simulink model "CoolingSystemR2024a_testingl"  (R2024a)
settings: Solver=ode1be  StartTime=0.0  StopTime=60*60  RelTol=1e-3
values from neighbouring files (symbols this model uses):
  cp = 4190    [parameters.m]
  M_B = 10000    [parameters.m]
  M_E = 2000    [parameters.m]
  M_MIX = 20    [parameters.m]
  mdot_ini = 30    [parameters.m]
  T_in = 60    [parameters.m]
  T_ini = 60    [parameters.m]
libraries: slpidlib x1
settings Model: ExtModeTrigDuration=100  Creator=mikman2  LastModifiedBy=ojklem
settings DataIOCC: StateSaveName=tmp_raccel_xout
settings OptimizationCC: EfficientMapNaN2IntZero=off
settings DebuggingCC: AlgebraicLoopMsg=error
settings RTWCC: CustomBLASCallback=coder.internal.blas.MATLABBLASCallback
settings CodeAppCC: GenerateComments=off  SimulinkBlockComments=off

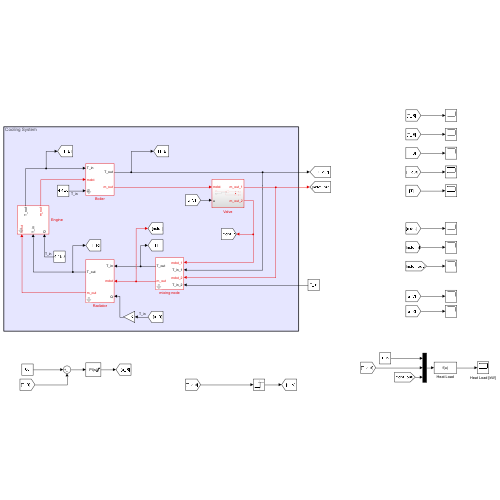
[thumbnail: Simulink's stored preview of the top-level diagram]
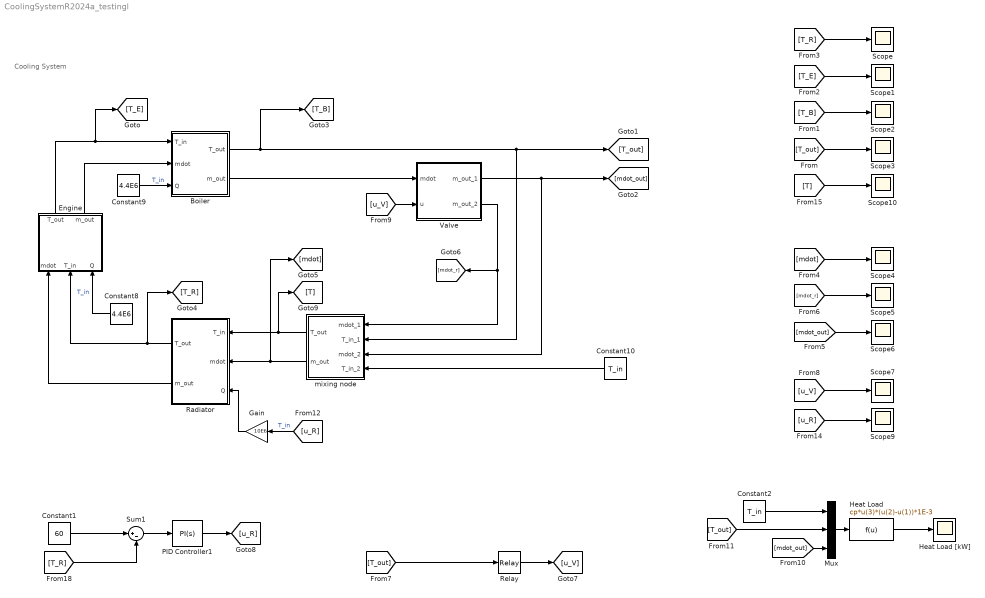
== system CoolingSystemR2024a_testingl ==
  note: Cooling System
  Boiler : Subsystem  mask{M=M_B, cp=cp}
      mask prompts: M "Mass [kg]"; cp "Specific heat capacity [J/kg/K]"
  Constant1 : Constant  Value=60
  Constant10 : Constant  Value=T_in
  Constant2 : Constant  Value=T_in
  Constant8 : Constant  Value=4.4E6
  Constant9 : Constant  Value=4.4E6
  Engine : Subsystem  mask{M=M_E, cp=cp}
      mask prompts: M "Mass [kg]"; cp "Specific heat capacity [J/kg/K]"
  Gain : Gain  Gain=10E6
  Heat Load : Fcn  Expr=cp*u(3)*(u(2)-u(1))*1E-3
  Heat Load [kW] : Scope
  Mux : Mux  Inputs=3
  PID Controller1 : slpidlib/PID Controller  Controller=PI  Form=Ideal  TimeDomain=Continuous-time  UseExternalTs=off  SampleTime=-1  IntegratorMethod=Forward Euler  FilterMethod=Forward Euler  ControllerParametersSource=internal  P=-0.05  I=1/120  UseKiTs=off  D=0  UseExternalDerivativeSource=off  N=100  UseFilter=on  TunerSelectOption=Transfer Function Based (PID Tuner App)  InitialConditionSource=internal  InitialConditionForIntegrator=0  InitialConditionForFilter=0  DifferentiatorICPrevScaledInput=0  ExternalReset=none  TrackingMode=off  Kt=1  LimitOutput=on  SatLimitsSource=internal  UpperSaturationLimit=1  LowerSaturationLimit=0  LinearizeAsGain=on  AntiWindupMode=none  Kb=1  LimitIntegrator=off  UpperIntegratorSaturationLimit=inf  LowerIntegratorSaturationLimit=-inf  POutMin=[]  POutMax=[]  IOutMin=[]  IOutMax=[]  DOutMin=[]  DOutMax=[]  NOutMin=[]  NOutMax=[]  SumOutMin=[]  SumOutMax=[]  SaturationOutMin=[]  SaturationOutMax=[]  PParamMin=[]  PParamMax=[]  IParamMin=[]  IParamMax=[]  DParamMin=[]  DParamMax=[]  NParamMin=[]  NParamMax=[]  KbParamMin=[]  KbParamMax=[]  KtParamMin=[]  KtParamMax=[]  KbOutMin=[]  KbOutMax=[]  KtOutMin=[]  KtOutMax=[]  IntegratorOutMin=[]  IntegratorOutMax=[]  FilterOutMin=[]  FilterOutMax=[]  SumI1OutMin=[]  SumI1OutMax=[]  SumI2OutMin=[]  SumI2OutMax=[]  SumI3OutMin=[]  SumI3OutMax=[]  SumI4OutMin=[]  SumI4OutMax=[]  SumDOutMin=[]  SumDOutMax=[]  DifferentiatorOutMin=[]  DifferentiatorOutMax=[]  FilterDiffOutCoefMin=[]  FilterDiffOutCoefMax=[]  ReciprocalOutMin=[]  ReciprocalOutMax=[]  SumDenOutMin=[]  SumDenOutMax=[]  SumNumOutMin=[]  SumNumOutMax=[]  DivideOutMin=[]  DivideOutMax=[]  UdiffTsProdOutMin=[]  UdiffTsProdOutMax=[]  NTsProdOutMin=[]  NTsProdOutMax=[]  UintegralTsProdOutMin=[]  UintegralTsProdOutMax=[]  UngainTsProdOutMin=[]  UngainTsProdOutMax=[]  ClampingZeroOutDataTypeStr=Inherit: Inherit via back propagation  ClampingZeroOutMin=[]  ClampingZeroOutMax=[]  FilterDenConstantOutDataTypeStr=Inherit: Inherit via back propagation  FilterDenConstantOutMin=[]  FilterDenConstantOutMax=[]  PCopyOutDataTypeStr=Inherit: Inherit via back propagation  PCopyOutMin=[]  PCopyOutMax=[]  NCopyOutDataTypeStr=Inherit: Inherit via back propagation  NCopyOutMin=[]  NCopyOutMax=[]  IntegratorContinuousStateAttributes=''  IntegratorStateMustResolveToSignalObject=off  IntegratorRTWStateStorageClass=Auto  FilterContinuousStateAttributes=''  FilterStateMustResolveToSignalObject=off  FilterRTWStateStorageClass=Auto  ParallelPVariant=Passthrough  IdealPVariant=InternalParameters  IVariant=InternalParameters  DVariant=Disabled  IntegratorVariant=Continuous  SatVariant=Enabled  AWVariant=Passthrough  PCopyVariant=Disabled  TRVariant=Disabled  FdbkBlocksVariant=Forward  IdealPFdbkVariant=Disabled  SatFdbkVariant=Disabled  DerivativeFilterVariant=Disabled  NVariant=Disabled  NCopyVariant=Disabled_SignalSpec  FilterICVariant=Disabled  IntegratorICVariant=InternalICs  ExternalResetVariant=Disabled  TRSumVariant=Passthrough  SumFdbkVariant=Disabled  SumVariant=Sum_PI  TsampFilterVariant=InternalTs  TsampNgainVariant=Passthrough  TsampIntegralVariant=Disabled_SignalSpec  ExternalSaturationOutDataTypeStr=Inherit: Same as second input  DerivativeSourceVariant=Disabled
  Radiator : Subsystem  mask{M=M_E, cp=cp}
      mask prompts: M "Mass [kg]"; cp "Specific heat capacity [J/kg/K]"
  Relay : Relay  OnSwitchValue=125  OffSwitchValue=0
  Scope{,1..7,9..10} (10 alike) : Scope
  Sum1 : Sum  Inputs=|+-
  Valve : Subsystem
  mixing node : Subsystem  mask{M=M_MIX, cp=cp}
      mask prompts: M "Mass [kg]"; cp "Specific heat capacity [J/kg/K]"
  wires:
  mixing node/1(T_out) -> [T], Radiator/1(T_in)
  mixing node/2(m_out) -> [mdot], Radiator/2(mdot)
  [u_R] -> Gain/1  "T_in"
  Radiator/2(m_out) -> Engine/1(mdot)
  Radiator/1(T_out) -> [T_R], Engine/2(T_in)
  Constant8/1 -> Engine/3(Q)  "T_in"
  Engine/1(T_out) -> Boiler/1(T_in), [T_E]
  Engine/2(m_out) -> Boiler/2(mdot)
  Constant9/1 -> Boiler/3(Q)  "T_in"
  Boiler/1(T_out) -> [T_B], mixing node/2(T_in_1), [T_out]
  Valve/1(m_out_1) -> [mdot_out], mixing node/3(mdot_2)
  Constant10/1 -> mixing node/4(T_in_2)
  Valve/2(m_out_2) -> mixing node/1(mdot_1), [mdot_r]
  Boiler/2(m_out) -> Valve/1(mdot)
  [u_V] -> Valve/2(u)
  [T_R] -> Scope/1
  [T_B] -> Scope2/1
  [T_E] -> Scope1/1
  [T_out] -> Scope3/1
  [mdot] -> Scope4/1
  [mdot_r] -> Scope5/1
  [mdot_out] -> Scope6/1
  [u_V] -> Scope7/1
  Gain/1 -> Radiator/3(Q)
  [u_R] -> Scope9/1
  [T] -> Scope10/1
  [T_out] -> Relay/1
  Relay/1 -> [u_V]
  Mux/1 -> Heat Load/1
  [mdot_out] -> Mux/3
  Constant2/1 -> Mux/1
  [T_out] -> Mux/2
  Heat Load/1 -> Heat Load [kW]/1
  Sum1/1 -> PID Controller1/1
  [T_R] -> Sum1/2
  Constant1/1 -> Sum1/1
  PID Controller1/1 -> [u_R]

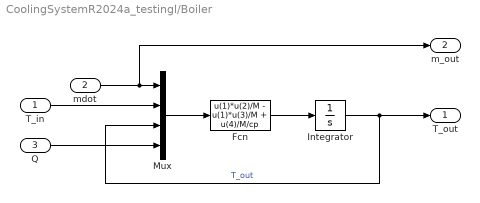
== system CoolingSystemR2024a_testingl/Boiler ==
  T_in : Inport
  mdot : Inport  Port=2
  Q : Inport  Port=3
  Fcn : Fcn  Expr=u(1)*u(2)/M - u(1)*u(3)/M + u(4)/M/cp
  Integrator : Integrator  InitialCondition=T_ini
  Mux : Mux
  T_out : Outport
  m_out : Outport  Port=2
  wires:
  Q/1 -> Mux/4
  T_in/1 -> Mux/2
  Mux/1 -> Fcn/1
  Fcn/1 -> Integrator/1
  mdot/1 -> m_out/1, Mux/1
  Integrator/1 -> T_out/1, Mux/3  "T_out"

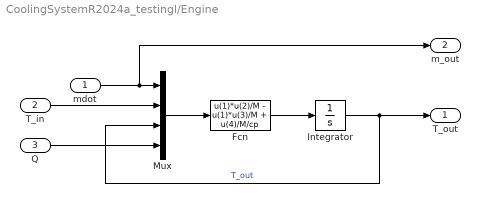
== system CoolingSystemR2024a_testingl/Engine ==
  mdot : Inport
  T_in : Inport  Port=2
  Q : Inport  Port=3
  Fcn : Fcn  Expr=u(1)*u(2)/M - u(1)*u(3)/M + u(4)/M/cp
  Integrator : Integrator  InitialCondition=T_ini
  Mux : Mux
  T_out : Outport
  m_out : Outport  Port=2
  wires:
  Integrator/1 -> Mux/3, T_out/1  "T_out"
  mdot/1 -> Mux/1, m_out/1
  Fcn/1 -> Integrator/1
  Mux/1 -> Fcn/1
  T_in/1 -> Mux/2
  Q/1 -> Mux/4

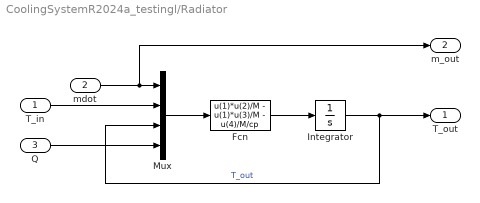
== system CoolingSystemR2024a_testingl/Radiator ==
  T_in : Inport
  mdot : Inport  Port=2
  Q : Inport  Port=3
  Fcn : Fcn  Expr=u(1)*u(2)/M - u(1)*u(3)/M - u(4)/M/cp
  Integrator : Integrator  InitialCondition=T_ini
  Mux : Mux
  T_out : Outport
  m_out : Outport  Port=2
  wires:
  Integrator/1 -> Mux/3, T_out/1  "T_out"
  mdot/1 -> Mux/1, m_out/1
  Fcn/1 -> Integrator/1
  Mux/1 -> Fcn/1
  T_in/1 -> Mux/2
  Q/1 -> Mux/4

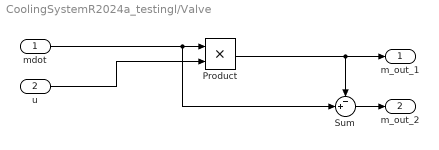
== system CoolingSystemR2024a_testingl/Valve ==
  mdot : Inport
  u : Inport  Port=2
  Product : Product
  Sum : Sum  Inputs=-+|
  m_out_1 : Outport
  m_out_2 : Outport  Port=2
  wires:
  mdot/1 -> Sum/2, Product/1
  Product/1 -> Sum/1, m_out_1/1
  u/1 -> Product/2
  Sum/1 -> m_out_2/1

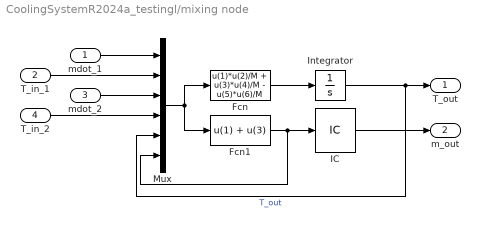
== system CoolingSystemR2024a_testingl/mixing node ==
  mdot_1 : Inport
  T_in_1 : Inport  Port=2
  mdot_2 : Inport  Port=3
  T_in_2 : Inport  Port=4
  Fcn : Fcn  Expr=u(1)*u(2)/M + u(3)*u(4)/M - u(5)*u(6)/M
  Fcn1 : Fcn  Expr=u(1) + u(3)
  IC : InitialCondition  Value=mdot_ini
  Integrator : Integrator  InitialCondition=T_ini
  Mux : Mux  Inputs=6
  T_out : Outport
  m_out : Outport  Port=2
  wires:
  Fcn1/1 -> IC/1, Mux/6
  T_in_2/1 -> Mux/4
  mdot_2/1 -> Mux/3
  T_in_1/1 -> Mux/2
  Mux/1 -> Fcn/1, Fcn1/1
  Fcn/1 -> Integrator/1
  mdot_1/1 -> Mux/1
  Integrator/1 -> T_out/1, Mux/5  "T_out"
  IC/1 -> m_out/1
